simulink model "mpc_ObstacleAvoidance"  (R2022b)
settings: Solver=VariableStepAuto  StartTime=0.0  StopTime=30  MaxStep=1e-3  RelTol=1e-3  EnableMultiTasking=on
values from neighbouring files (symbols this model uses):
  eps_0 = [0 ... (first row only)    [main_nonlin.m]    (also in maina.m; maina_theirs.m; qwdui.m; ref_tracking.m = [0;0;0;0.9*V])
  lanes = 3    [main_nonlin.m]    (also in maina.m; maina_theirs.m; qwdui.m; ref_tracking.m)
  lanewidth = 3.5    [main_nonlin.m]    (also in maina.m; maina_theirs.m; qwdui.m; ref_tracking.m)
  obstacle = struct    [ObstacleParametersforMain.m]    (also in createObstacle.m = ObstacleGeometry(obstacle); main_nonlin.m = createObstacle(); maina_theirs.m = createObstacle(); qwdui.m = createObstacle())
  parameters = [m;I;a;b]    [main_nonlin.m]    (also in maina.m = [m;I;a;b;c]; maina_theirs.m = [m;I;a;b;c]; qwdui.m = [m;I;a;b;c]; ref_tracking.m = [m;I;a;b;c])
  u_0 = ones(3,1)    [main_nonlin.m]    (also in maina.m = zeros(5,1); maina_theirs.m; qwdui.m = zeros(5,1); ref_tracking.m = zeros(2,1))
  V = eps(4)    [linearSS.m]    (also in main_nonlin.m = 10; maina.m = 13.8888888889; maina_theirs.m = 20; qwdui.m = 20)
libraries: mpclib x1
settings Model: Creator=The MathWorks, Inc.  LastModifiedBy=Givani
settings SolverCC: AlgebraicLoopSolver=LineSearch  MinimalZcImpactIntegration=on
settings DataIOCC: LimitDataPoints=on  SaveFormat=Array  SaveOutput=off  DSMLogging=off  SaveTime=off  ReturnWorkspaceOutputs=off
settings OptimizationCC: LifeSpan=inf
settings DebuggingCC: AlgebraicLoopMsg=none  UnderspecifiedInitializationDetection=Classic  MergeDetectMultiDrivingBlocksExec=none  SolverPrmCheckMsg=warning  UnconnectedInputMsg=warning  UnconnectedOutputMsg=warning  UnconnectedLineMsg=warning  AllowSymbolicDim=off  StateNameClashWarn=warning  SFUnexpectedBacktrackingDiag=warning  SFNoUnconditionalDefaultTransitionDiag=warning  SFExecutionAtInitializationDiag=none  SFMachineParentedDataDiag=warning  ArithmeticOperatorsInVariantConditions=warning
settings HardwareCC: ProdBitPerPointer=32  ProdBitPerSizeT=32  ProdBitPerPtrDiffT=32  ProdLargestAtomicFloat=None  ProdIntDivRoundTo=Undefined  ProdEndianess=Unspecified  ProdWordSize=32  ProdHWDeviceType=32-bit Generic
settings ModelReferenceCC: EnableRefExpFcnMdlSchedulingChecks=on  PropagateSignalLabelsOutOfModel=off
settings SFSimCC: SimUseLocalCustomCode=off  CustomCodeUndefinedFunction=UseInterfaceOnly
settings RTWCC: RTWUseLocalCustomCode=off
settings CodeAppCC: StateflowObjectComments=on
settings GRTTargetCC: TargetLangStandard=C89/C90 (ANSI)
settings ConfigComp: CovMetricSettings=dw  CovSaveCumulativeToWorkspaceVar=on  CovSaveSingleToWorkspaceVar=on  CovExternalEMLEnable=off  CovSFcnEnable=off
settings SimscapeCC: SimscapeNormalizeSystem=off  SimscapeNominalValues="[{\"value\":\"10\",\"unit\":\"V\"},{\"value\":\"1\",\"unit\":\"A\"},{\"value\":\"10\",\"unit\":\"N*m\"},{\"value\":\"10\",\"unit\":\"bar\"},{\"value\":\"100\",\"unit\":\"kJ/kg\"},{\"value\":\"1\",\"unit\":\"kW\"},{\"value\":\"300\",\"unit\":\"K\"},{\"value\":\"100\",\"unit\":\"cm^3/s\"},{\"value\":\"1\",\"unit\":\"kN\"},{\"value\":\"1\",\"unit\":\"g/cm^3\"},{\"value\":\"1\",\"unit\":\"l\"},{\"value\":\"1\",\"unit\":\"cm^2\"},{\"value\":\"60\",\"unit\":\"Hz\"}]"
settings ConfigurationSet: Description=SimMechanics 2G
settings ExplorerConfigSet: InternalSimMechanicsExplorerSettings="<ExplorerConfiguration><canonicalview>default</canonicalview><AnimationSetting><BasePlaybackSpeed>1.0</BasePlaybackSpeed><PlaybackSpeedFactor>1.0</PlaybackSpeedFactor></AnimationSetting><TilePanel><TileInfo><Tiles Columns=\"1\" Count=\"1\" Rows=\"1\"><Column Left=\"2\" Weight=\"1\"/><Column Left=\"1552\"/><Row Top=\"2\" Weight=\"1\"/><Row Top=\"932\"/><Tile Height=\"1\" Width=\"1\" X=\"0\" Y=\"0\"/></Tiles></TileInfo><SceneInfo><SceneViewer><BGColor><R>0.60000002384185791</R><G>0.60000002384185791</G><B>0.60000002384185791</B></BGColor><Camera><Position><X>0.027865189060748197</X><Y>-2.5719092456962986</Y><Z>0.23157896538506753</Z></Position><Center><X>0.62659712312732463</X><Y>-0.46110119691712204</Y><Z>0.22087365386473376</Z></Center><Up><X>-0.0079438354874226333</X><Y>0.0073246425924307582</Y><Z>0.99994162084025784</Z></Up><Left>-0.24533778208815546</Left><Right>0.24533778208815546</Right><Bottom>-0.79734779727023208</Bottom><Top>0.79734779727023208</Top></Camera></SceneViewer></SceneInfo></TilePanel></ExplorerConfiguration>"

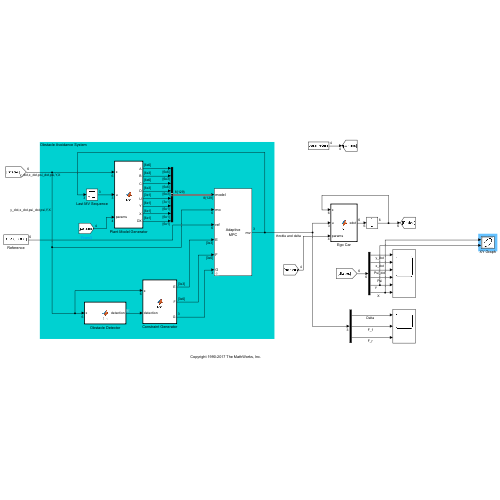
[thumbnail: Simulink's stored preview of the top-level diagram]
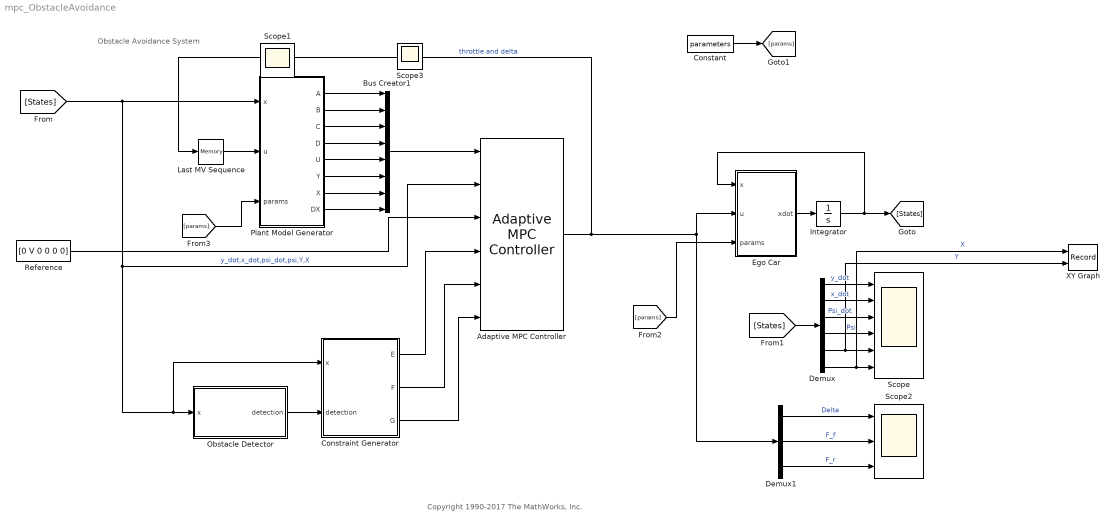
== system mpc_ObstacleAvoidance ==
  note: Obstacle Avoidance System
  note: Copyright 1990-2017 The MathWorks, Inc.
  Adaptive MPC Controller : mpclib/Adaptive MPC Controller  SCDEnableBlockLinearizationSpecification=on  mpcobj=mpcobj  enable_value=0  updateMPCinCallerWorkspace=on  md_inport=off  mv_inport=off  uref_inport=off  return_cost=off  return_mvseq=off  return_qpstatus=off  return_xseq=off  return_state=off  return_ovseq=off  state_inport=off  isltv_plant=off  umin_inport=off  umax_inport=off  ymin_inport=off  ymax_inport=off  cc_inport=on  ywt_inport=off  uwt_inport=off  duwt_inport=off  rhoeps_inport=off  pm_inport=off  MaximumP=10  HorizonChoice=FixedHorizon  BlockDataType=double  SampleTimeInherited=off  switch_inport=off
  Bus Creator1 : BusCreator  Inputs=8
  Constant : Constant  Value=parameters
  Constraint Generator : MATLAB Function  TreatAsAtomicUnit=on
  Demux : Demux  Outputs=6
  Demux1 : Demux  Outputs=3
  Ego Car : MATLAB Function  TreatAsAtomicUnit=on
  Integrator : Integrator  InitialCondition=eps_0
  Last MV Sequence : Memory  InitialCondition=u_0  InheritSampleTime=on
  Obstacle Detector : MATLAB Function  TreatAsAtomicUnit=on
  Plant Model Generator : MATLAB Function  TreatAsAtomicUnit=on
  Reference : Constant  Value=[0 V 0 0 0 0]
  Scope : Scope  NumInputPorts=6
  Scope2 : Scope  NumInputPorts=3
  XY Graph : Record  FileSettingsInternal="{\"entries\":[{\"content\":{\"excelSettings\":{\"content\":{},\"type\":\"Streamout.ExcelSettings\"}},\"type\":\"Streamout.FileSettingStorage\",\"uuid\":\"310cba75-c626-4fed-9bba-b2bcbd072042\"}],\"packageUris\":[\"http://schema.mathworks.com/mf0/streamout_blocks/R2020a\"],\"version\":\"1.0\"}"  Layout=[1 1]  SignalsInternal="{\"entries\":[{\"content\":{\"signals\":[{\"content\":{\"blockPath\":[\"mpc_ObstacleAvoidance/XY Graph\"],\"channel\":[],\"dimensions\":[1],\"domain\":\"mpc_ObstacleAvoidance/XY Graph\",\"lineColor\":\"#a2142f\",\"plots\":[1],\"port\":1,\"sid\":[\"\"],\"signalID\":380,\"signalName\":\"X\"},\"type\":\"RecordBlkView.Signal\",\"uuid\":\"442a5daf-36a9-48a2-ac0c-bda2413994db\"},{\"content\":{\"blockPath\":[\"mpc_ObstacleAvoidance/XY Graph\"],\"channel\":[],\"dimensions\":[1],\"domain\":\"mpc_ObstacleAvoidance/XY Graph\",\"lineColor\":\"#139fff\",\"plots\":[1],\"port\":2,\"sid\":[\"\"],\"signalID\":384,\"signalName\":\"Y\"},\"type\":\"RecordBlkView.Signal\",\"uuid\":\"2c062c61-8883-47aa-bf24-cdee08f7816e\"}]},\"type\":\"RecordBlkView.InputSignals\",\"uuid\":\"5e0df64b-097e-4499-acec-f71161c01be6\"}],\"packageUris\":[\"http://schema.mathworks.com/mf0/streamout_blocks/R2020a\"],\"version\":\"1.0\"}"  VisualizationBindings="{\"xyplotplugin\":{\"info\":[{\"series\":[{\"bindingParametersList\":[{\"parameter\":\"X-Axis\",\"signalID\":380,\"signalName\":\"X\"},{\"parameter\":\"Y-Axis\",\"signalID\":384,\"signalName\":\"Y\"}],\"seriesID\":57730}],\"subplotID\":1}]}}"  CompatibilityTag=XY
  Scope1 : Scope
  Scope3 : Scope
  wires:
  Demux/4 -> Scope/4  "Psi"
  Demux/3 -> Scope/3  "Psi_dot"
  Demux/2 -> Scope/2  "x_dot"
  Demux/1 -> Scope/1  "y_dot"
  Bus Creator1/1 -> Adaptive MPC Controller/1
  Last MV Sequence/1 -> Plant Model Generator/2(u)
  Reference/1 -> Adaptive MPC Controller/3
  Plant Model Generator/1(A) -> Bus Creator1/1
  Plant Model Generator/2(B) -> Bus Creator1/2
  Plant Model Generator/3(C) -> Bus Creator1/3
  Plant Model Generator/4(D) -> Bus Creator1/4
  Plant Model Generator/5(U) -> Bus Creator1/5
  Plant Model Generator/6(Y) -> Bus Creator1/6
  Plant Model Generator/7(X) -> Bus Creator1/7
  Plant Model Generator/8(DX) -> Bus Creator1/8
  Integrator/1 -> [States], Ego Car/1(x)
  Adaptive MPC Controller/1 -> Ego Car/2(u), Demux1/1, Last MV Sequence/1  "throttle and delta"
  Ego Car/1(xdot) -> Integrator/1
  [States] -> Demux/1
  [States] -> Adaptive MPC Controller/2, Obstacle Detector/1(x), Constraint Generator/1(x), Plant Model Generator/1(x)  "y_dot,x_dot,psi_dot,psi,Y,X"
  Obstacle Detector/1(detection) -> Constraint Generator/2(detection)
  Constraint Generator/1(E) -> Adaptive MPC Controller/4
  Constraint Generator/2(F) -> Adaptive MPC Controller/5
  Constraint Generator/3(G) -> Adaptive MPC Controller/6
  Demux1/1 -> Scope2/1  "Delta"
  Demux1/2 -> Scope2/2  "F_f"
  [params] -> Ego Car/3(params)
  Constant/1 -> [params]
  [params] -> Plant Model Generator/3(params)
  Demux/5 -> XY Graph/2, Scope/5  "Y"
  Demux/6 -> XY Graph/1, Scope/6  "X"
  Demux1/3 -> Scope2/3  "F_r"

== matlab function mpc_ObstacleAvoidance/Ego Car ==
  settings: updateMethod=DISCRETE  sampleTime=Ts
  data: x input; u input; xdot output; params input
function xdot = fcn(x,u,params)
xdot = LTIC(x,u,params);

== matlab function mpc_ObstacleAvoidance/Plant Model Generator ==
  settings: updateMethod=DISCRETE  sampleTime=Ts
  data: x input size=[6,1]; u input size=[3,1]; A output size=[6,6]; B output size=[6,3]; C output size=[6,6]; D output; U output size=[3,1]; Y output size=[6, 1]; X output size=[6,1]; DX output size=[6,1]; Ts parameter; params input size=[4,1]
function [A,B,C,D,U,Y,X,DX] = fcn(x,u,Ts, params)

[A,B,C,D,U,Y,X,DX] = discreteSS_simulink(x,u,params,Ts);

== matlab function mpc_ObstacleAvoidance/Obstacle Detector ==
  settings: updateMethod=DISCRETE  sampleTime=Ts
  data: x input; obstacle parameter; detection output
function detection  = fcn(x,obstacle)
% Detection Logic: it determine when the vehicle sees the obstacle
detection = ObstacleDetect(x,obstacle);

== matlab function mpc_ObstacleAvoidance/Constraint Generator ==
  settings: updateMethod=DISCRETE  sampleTime=Ts
  data: x input; detection input; obstacle parameter; lanewidth parameter; E output; F output; G output; lanes parameter
function [E,F,G] = fcn(x,detection,obstacle,lanewidth,lanes)
% Generate run-time custom constraint
[E,F,G] = updateConstraints(x,obstacle,detection,lanewidth,lanes);
